simulink model "Project_sim"  (R2024a)
settings: Solver=FixedStepAuto  StartTime=0.0  StopTime=0.05  FixedStep=5e-05  RelTol=1e-3
libraries: spsRMSLib x4, spsThreePhaseFaultLib x3, spsThreePhaseSourceLib x3, spsThreePhasePISectionLineLib x2, spsThreePhaseTransformerTwoWindingsLib x2, spsThreePhaseVIMeasurementLib x2, spsThreePhaseBreakerLib x2, spsThreePhaseSeriesRLCLoadLib x1, spspowerguiLib x1
settings Model: Creator=am.en.u4eee22052  LastModifiedBy=Achuoth Akol Achuoth
settings DataIOCC: SaveFormat=StructureWithTime  SaveOutput=off  SignalLogging=off  DSMLogging=off  SaveTime=off  ReturnWorkspaceOutputs=off

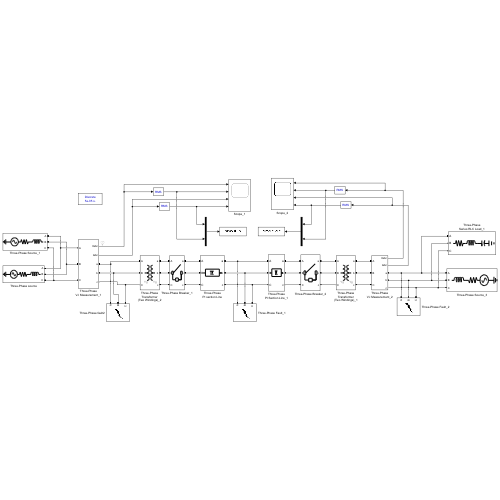
[thumbnail: Simulink's stored preview of the top-level diagram]
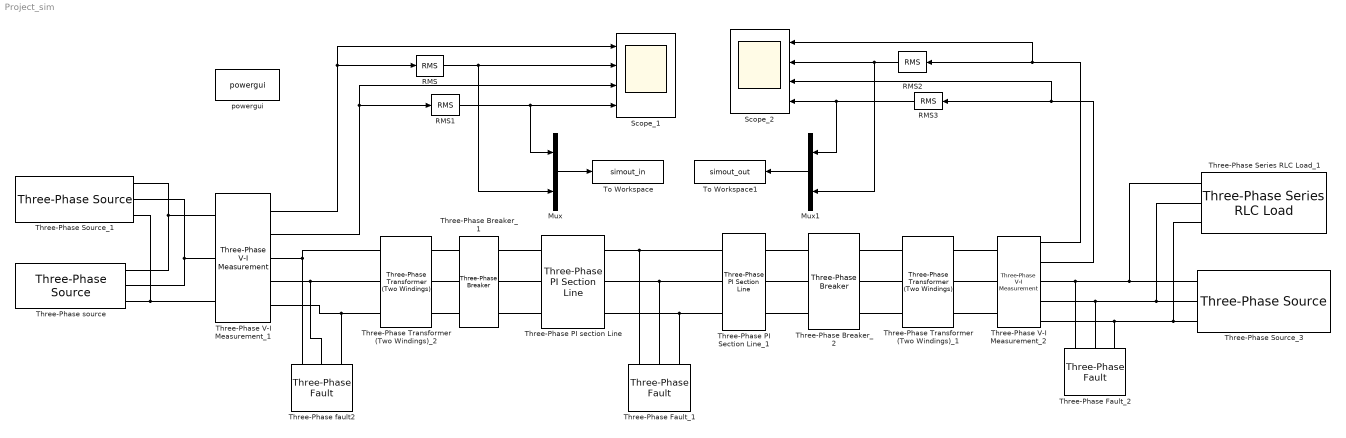
== system Project_sim ==
  Mux : Mux  Inputs=2
  Mux1 : Mux  Inputs=2
  RMS{,1..3} (4 alike) : spsRMSLib/RMS  TrueRMS=on  Freq=50  RMSInit=0  Ts=0.001
  Scope_1 : Scope  NumInputPorts=4
  Scope_2 : Scope  NumInputPorts=4
  Three-Phase PI Section Line_1 : spsThreePhasePISectionLineLib/Three-Phase PI Section Line  LConnTagsString=a|b|c  RConnTagsString=A|B|C  Length=300  Frequency=50  Resistances=[0.01273 0.3864]  Inductances=[0.9337e-3 4.1264e-3]  Capacitances=[12.74e-9 7.751e-9]
  Three-Phase PI section Line : spsThreePhasePISectionLineLib/Three-Phase PI Section Line  LConnTagsString=a|b|c  RConnTagsString=A|B|C  Length=300  Frequency=50  Resistances=[0.01273 0.3864]  Inductances=[1.0e-3 4.0e-3]  Capacitances=[13e-9 8e-9]
  Three-Phase Series RLC Load_1 : spsThreePhaseSeriesRLCLoadLib/Three-Phase Series RLC Load  LConnTagsString=A|B|C  Configuration=Y (grounded)  NominalVoltage=1000  Vabc=[1e3 1e3 1e3]  Vabcp=[1e3 1e3 1e3]  NominalFrequency=50  UnbalancedPower=off  ActivePower=10e3  InductivePower=100  CapacitivePower=100  Pabc=[10e3 9e3 11e3]  QLabc=[100 90 110]  QCabc=[100 90 110]  Pabcp=[10e3 9e3 11e3]  QLabcp=[100 90 110]  QCabcp=[100 90 110]  Measurements=None  LoadType=constant Z
  Three-Phase Transformer (Two Windings)_1 : spsThreePhaseTransformerTwoWindingsLib/Three-Phase Transformer (Two Windings)  Winding1Connection=Yg  Winding2Connection=Yg  CoreType=Three single-phase transformers  SetSaturation=off  Hysteresis=off  DataFile='hysteresis'  SetInitialFlux=off  Measurements=None  UNITS=pu  NominalPower=[ 1e3 , 50 ]  Winding1=[ 11e3 , 0.002 , 0.08 ]  Winding2=[ 0.4e3 , 0.002 , 0.08 ]  Rm=500  Lm=500  L0=0.5  Saturation=[ 0,0 ; 0.0024,1.2 ; 1.0,1.52 ]  InitialFluxes=[-0.00998217708121243 0.00491418069430346 0.00506799638690897]  BreakLoop=on  DiscreteSolver=Trapezoidal iterative  DataType=off  TransfoNumber=1
  Three-Phase Transformer (Two Windings)_2 : spsThreePhaseTransformerTwoWindingsLib/Three-Phase Transformer (Two Windings)  Winding1Connection=Yg  Winding2Connection=Yg  CoreType=Three single-phase transformers  SetSaturation=off  Hysteresis=off  DataFile='hysteresis'  SetInitialFlux=off  Measurements=None  UNITS=pu  NominalPower=[ 1e3 , 50 ]  Winding1=[ 11e3 , 0.002 , 0.08 ]  Winding2=[ 0.4e3 , 0.002 , 0.08 ]  Rm=500  Lm=500  L0=0.5  Saturation=[ 0,0 ; 0.0024,1.2 ; 1.0,1.52 ]  InitialFluxes=[-0.966327725148709 0.586663286633682 0.379664438515027]  BreakLoop=on  DiscreteSolver=Trapezoidal iterative  DataType=off  TransfoNumber=1
  Three-Phase V-I Measurement_1 : spsThreePhaseVIMeasurementLib/Three-Phase V-I Measurement  VoltageMeasurement=phase-to-ground  SetLabelV=off  LabelV=Vabc  Vpu=off  VpuLL=off  CurrentMeasurement=yes  SetLabelI=off  LabelI=Iabc  Ipu=off  Pbase=100e6  Vbase=500e3  OutputType=Complex  PhasorSimulation=off  PSBequivalent=0
  Three-Phase V-I Measurement_2 : spsThreePhaseVIMeasurementLib/Three-Phase V-I Measurement  VoltageMeasurement=phase-to-ground  SetLabelV=off  LabelV=Vabc  Vpu=off  VpuLL=off  CurrentMeasurement=yes  SetLabelI=off  LabelI=Iabc  Ipu=off  Pbase=100e6  Vbase=500e3  OutputType=Complex  PhasorSimulation=off  PSBequivalent=0
  Three-Phase Breaker_1 : spsThreePhaseBreakerLib/Three-Phase Breaker  InitialState=open  SwitchA=on  SwitchB=on  SwitchC=on  SwitchTimes=[3/50]  External=off  BreakerResistance=0.01  SnubberResistance=1e6  SnubberCapacitance=inf  Measurements=None
  Three-Phase Breaker_2 : spsThreePhaseBreakerLib/Three-Phase Breaker  InitialState=open  SwitchA=on  SwitchB=on  SwitchC=on  SwitchTimes=[3/50]  External=off  BreakerResistance=0.01  SnubberResistance=1e6  SnubberCapacitance=inf  Measurements=None
  Three-Phase Fault_1 : spsThreePhaseFaultLib/Three-Phase Fault  InitialStates=0  FaultA=off  FaultB=off  FaultC=off  GroundFault=off  SwitchTimes=[0.029106 0.062743]  External=off  SwitchStatus=NaN  FaultResistance=50  GroundResistance=0.048827  SnubberResistance=1e6  SnubberCapacitance=inf  Measurements=None
  Three-Phase Fault_2 : spsThreePhaseFaultLib/Three-Phase Fault  InitialStates=0  FaultA=off  FaultB=off  FaultC=off  GroundFault=off  SwitchTimes=[0.020760 0.055558]  External=off  SwitchStatus=NaN  FaultResistance=50  GroundResistance=0.046163  SnubberResistance=1e6  SnubberCapacitance=inf  Measurements=None
  Three-Phase Source_1 : spsThreePhaseSourceLib/Three-Phase Source  InternalConnection=Yg  VoltagePhases=off  Voltage=11e3  PhaseAngle=30  Voltage_phases=[25e3 25e3 25e3]/sqrt(3)  PhaseAngles_phases=[0 -120 +120]  Frequency=50  NonIdealSource=on  SpecifyImpedance=on  Resistance=0.52176  Inductance=0.0032472  ShortCircuitLevel=30e6  BaseVoltage=11e3  XRratio=7  BusType=swing  Pref=10e3  Qref=0  Prefabc=[10e3, 10e3, 10e3]  Qrefabc=[0, 0, 0]  Qmin=-inf  Qmax=inf
  Three-Phase Source_3 : spsThreePhaseSourceLib/Three-Phase Source  InternalConnection=Yg  VoltagePhases=off  Voltage=11e3  PhaseAngle=30  Voltage_phases=[25e3 25e3 25e3]/sqrt(3)  PhaseAngles_phases=[0 -120 +120]  Frequency=50  NonIdealSource=on  SpecifyImpedance=on  Resistance=0.8929  Inductance=16.58e-3  ShortCircuitLevel=30e6  BaseVoltage=11e3  XRratio=7  BusType=swing  Pref=10e3  Qref=0  Prefabc=[10e3, 10e3, 10e3]  Qrefabc=[0, 0, 0]  Qmin=-inf  Qmax=inf
  Three-Phase fault2 : spsThreePhaseFaultLib/Three-Phase Fault  InitialStates=0  FaultA=on  FaultB=on  FaultC=on  GroundFault=on  SwitchTimes=[0.021450 0.068510]  External=off  SwitchStatus=NaN  FaultResistance=50  GroundResistance=0.059487  SnubberResistance=1e6  SnubberCapacitance=inf  Measurements=None
  Three-Phase source : spsThreePhaseSourceLib/Three-Phase Source  InternalConnection=Yg  VoltagePhases=off  Voltage=11e3  PhaseAngle=30  Voltage_phases=[25e3 25e3 25e3]/sqrt(3)  PhaseAngles_phases=[0 -120 +120]  Frequency=50  NonIdealSource=on  SpecifyImpedance=on  Resistance=0.8929  Inductance=16.58e-3  ShortCircuitLevel=30e6  BaseVoltage=11e3  XRratio=7  BusType=swing  Pref=10e3  Qref=0  Prefabc=[10e3, 10e3, 10e3]  Qrefabc=[0, 0, 0]  Qmin=-inf  Qmax=inf
  To Workspace : ToWorkspace  VariableName=simout_in  SaveFormat=Structure With Time  SampleTime=-1
  To Workspace1 : ToWorkspace  VariableName=simout_out  SaveFormat=Structure With Time  SampleTime=-1
  powergui : spspowerguiLib/powergui  Priority=1  SimulationMode=Discrete  SampleTime=5e-5  frequency=60  Iterations=50  frequencyindice=50  Pbase=100e6  ErrMax=1e-4  UnitsV=kV  UnitsW=MW  buscounter=0  FunctionMessages=off  echomessages=off  EnableUseOfTLC=off  CurrentSourceSwitches=off  DisableSnubberDevices=off  DisableRonSwitches=off  DisableVfSwitches=off  DisplayEquations=off  AutomaticDiscreteSolvers=off  SolverType=Tustin/Backward Euler (TBE)  Interpol=off  ExternalGateDelay=off  methode=off  Ts=100  x0status=blocks  SPID=on  SwTol=0  HookPort=off  NonlinearTolerance=1e-4  nMaxIteration=100  ContinueOnMaxIteration=off  RestoreLinks=warning  ResistiveCurrentMeasurement=off  Frange=[0:2:500]  Ylog=off  Xlog=on  ShowGrid=off  save=off  variable=ZData  structure=0  ZoomFFT=off  StartTime=0.0  cycles=1  DisplayStyle=1  fundamental=60  FreqAxis=off  MaxFrequency=1000  frequencyindicesteady=1  RmsSteady=1  display=off
  wires:
  Three-Phase V-I Measurement_2/1 -> Scope_2/1, RMS2/1
  Three-Phase V-I Measurement_2/2 -> Scope_2/3, RMS3/1
  Mux1/1 -> To Workspace1/1
  Mux/1 -> To Workspace/1
  Three-Phase V-I Measurement_1/2 -> Scope_1/3, RMS1/1
  Three-Phase V-I Measurement_1/1 -> Scope_1/1, RMS/1
  RMS1/1 -> Mux/1, Scope_1/4
  RMS/1 -> Mux/2, Scope_1/2
  RMS2/1 -> Scope_2/2, Mux1/2
  RMS3/1 -> Mux1/1, Scope_2/4
  connections:
  Three-Phase V-I Measurement_1/LConn1 -- Three-Phase source/RConn1 -- Three-Phase Source_1/RConn1
  Three-Phase V-I Measurement_1/LConn2 -- Three-Phase source/RConn2 -- Three-Phase Source_1/RConn2
  Three-Phase V-I Measurement_1/LConn3 -- Three-Phase source/RConn3 -- Three-Phase Source_1/RConn3
  Three-Phase Transformer (Two Windings)_2/LConn2 -- Three-Phase fault2/LConn2 -- Three-Phase V-I Measurement_1/RConn2
  Three-Phase Transformer (Two Windings)_2/LConn3 -- Three-Phase V-I Measurement_1/RConn3 -- Three-Phase fault2/LConn3
  Three-Phase V-I Measurement_1/RConn1 -- Three-Phase Transformer (Two Windings)_2/LConn1 -- Three-Phase fault2/LConn1
  Three-Phase Breaker_1/LConn1 -- Three-Phase Transformer (Two Windings)_2/RConn1
  Three-Phase Transformer (Two Windings)_2/RConn2 -- Three-Phase Breaker_1/LConn2
  Three-Phase Transformer (Two Windings)_2/RConn3 -- Three-Phase Breaker_1/LConn3
  Three-Phase Breaker_2/RConn1 -- Three-Phase Transformer (Two Windings)_1/LConn1
  Three-Phase Transformer (Two Windings)_1/LConn2 -- Three-Phase Breaker_2/RConn2
  Three-Phase Breaker_2/RConn3 -- Three-Phase Transformer (Two Windings)_1/LConn3
  Three-Phase V-I Measurement_2/LConn1 -- Three-Phase Transformer (Two Windings)_1/RConn1
  Three-Phase Transformer (Two Windings)_1/RConn2 -- Three-Phase V-I Measurement_2/LConn2
  Three-Phase Transformer (Two Windings)_1/RConn3 -- Three-Phase V-I Measurement_2/LConn3
  Three-Phase V-I Measurement_2/RConn1 -- Three-Phase Fault_2/LConn1 -- Three-Phase Series RLC Load_1/LConn1 -- Three-Phase Source_3/RConn1
  Three-Phase V-I Measurement_2/RConn2 -- Three-Phase Fault_2/LConn2 -- Three-Phase Series RLC Load_1/LConn2 -- Three-Phase Source_3/RConn2
  Three-Phase Fault_2/LConn3 -- Three-Phase Series RLC Load_1/LConn3 -- Three-Phase Source_3/RConn3 -- Three-Phase V-I Measurement_2/RConn3
  Three-Phase Breaker_1/RConn1 -- Three-Phase PI section Line/LConn1
  Three-Phase Breaker_1/RConn2 -- Three-Phase PI section Line/LConn2
  Three-Phase Breaker_1/RConn3 -- Three-Phase PI section Line/LConn3
  Three-Phase PI Section Line_1/RConn3 -- Three-Phase Breaker_2/LConn3
  Three-Phase PI Section Line_1/LConn3 -- Three-Phase PI section Line/RConn3 -- Three-Phase Fault_1/LConn3
  Three-Phase PI section Line/RConn2 -- Three-Phase Fault_1/LConn2 -- Three-Phase PI Section Line_1/LConn2
  Three-Phase PI Section Line_1/RConn2 -- Three-Phase Breaker_2/LConn2
  Three-Phase PI Section Line_1/RConn1 -- Three-Phase Breaker_2/LConn1
  Three-Phase PI section Line/RConn1 -- Three-Phase Fault_1/LConn1 -- Three-Phase PI Section Line_1/LConn1
